simulink model "Stateflow_code"  (R2020a)
settings: Solver=ode5  StartTime=0.0  StopTime=inf  FixedStep=0.01  RelTol=1e-3
StopFcn:
  | clear con
model workspace (MAT data in the model file):
  A : Simulink.Signal (value not decoded)
undefined symbols (not defined in the file or in its folder): sigbuilder_block
libraries: simulink x10, simulink_extras x7, aerolibanimutils x1, powerlib_meascontrol x1, dspswit3 x1
(part 2 of 2)

== system Stateflow_code/Systemtest Simulation1/2_rot_mit_Deckel/luft_an ==
  Add : Sum
  Constant : Constant
  Constant1 : Constant  Value=-1
  Data Type Conversion : DataTypeConversion  OutDataTypeStr=boolean
  Delay : Delay  DelayLength=550
  Delay1 : Delay  DelayLength=750
  Out1 : Outport  VectorParamsAs1DForOutWhenUnconnected=off
  wires:
  Constant/1 -> Delay/1
  Constant1/1 -> Delay1/1
  Delay/1 -> Add/1
  Delay1/1 -> Add/2
  Add/1 -> Data Type Conversion/1
  Data Type Conversion/1 -> Out1/1

== system Stateflow_code/Systemtest Simulation1/2_rot_mit_Deckel/out5 ==
  Add : Sum
  Constant : Constant
  Constant1 : Constant  Value=-1
  Data Type Conversion : DataTypeConversion  OutDataTypeStr=boolean
  Delay : Delay  DelayLength=0
  Delay1 : Delay  DelayLength=0
  Out1 : Outport  VectorParamsAs1DForOutWhenUnconnected=off
  wires:
  Constant/1 -> Delay/1
  Constant1/1 -> Delay1/1
  Delay/1 -> Add/1
  Delay1/1 -> Add/2
  Add/1 -> Data Type Conversion/1
  Data Type Conversion/1 -> Out1/1

== system Stateflow_code/Systemtest Simulation1/2_rot_mit_Deckel/out6 ==
  Add : Sum
  Constant : Constant
  Constant1 : Constant  Value=-1
  Data Type Conversion : DataTypeConversion  OutDataTypeStr=boolean
  Delay : Delay  DelayLength=0
  Delay1 : Delay  DelayLength=0
  Out1 : Outport  VectorParamsAs1DForOutWhenUnconnected=off
  wires:
  Constant/1 -> Delay/1
  Constant1/1 -> Delay1/1
  Delay/1 -> Add/1
  Delay1/1 -> Add/2
  Add/1 -> Data Type Conversion/1
  Data Type Conversion/1 -> Out1/1

== system Stateflow_code/Systemtest Simulation1/2_rot_mit_Deckel/out7 ==
  Add : Sum
  Constant : Constant
  Constant1 : Constant  Value=-1
  Data Type Conversion : DataTypeConversion  OutDataTypeStr=boolean
  Delay : Delay  DelayLength=0
  Delay1 : Delay  DelayLength=0
  Out1 : Outport  VectorParamsAs1DForOutWhenUnconnected=off
  wires:
  Constant/1 -> Delay/1
  Constant1/1 -> Delay1/1
  Delay/1 -> Add/1
  Delay1/1 -> Add/2
  Add/1 -> Data Type Conversion/1
  Data Type Conversion/1 -> Out1/1

== system Stateflow_code/Systemtest Simulation1/2_rot_mit_Deckel/station_frei ==
  Add : Sum
  Constant : Constant
  Constant1 : Constant  Value=-1
  Data Type Conversion : DataTypeConversion  OutDataTypeStr=boolean
  Delay : Delay  DelayLength=0
  Delay1 : Delay  DelayLength=10
  Out1 : Outport  VectorParamsAs1DForOutWhenUnconnected=off
  wires:
  Constant/1 -> Delay/1
  Constant1/1 -> Delay1/1
  Delay/1 -> Add/1
  Delay1/1 -> Add/2
  Add/1 -> Data Type Conversion/1
  Data Type Conversion/1 -> Out1/1

== system Stateflow_code/Systemtest Simulation1/2_rot_mit_Deckel/zylinder_ausschieben ==
  Add : Sum
  Constant : Constant
  Constant1 : Constant  Value=-1
  Data Type Conversion : DataTypeConversion  OutDataTypeStr=boolean
  Delay : Delay  DelayLength=550
  Delay1 : Delay  DelayLength=620
  Out1 : Outport  VectorParamsAs1DForOutWhenUnconnected=off
  wires:
  Constant/1 -> Delay/1
  Constant1/1 -> Delay1/1
  Delay/1 -> Add/1
  Delay1/1 -> Add/2
  Add/1 -> Data Type Conversion/1
  Data Type Conversion/1 -> Out1/1

== system Stateflow_code/Systemtest Simulation1/2_rot_mit_Deckel/zylinder_entfernt_folge ==
  Add : Sum
  Constant : Constant
  Constant1 : Constant  Value=-1
  Data Type Conversion : DataTypeConversion  OutDataTypeStr=boolean
  Delay : Delay  DelayLength=1000
  Delay1 : Delay  DelayLength=1050
  Out1 : Outport  VectorParamsAs1DForOutWhenUnconnected=off
  wires:
  Constant/1 -> Delay/1
  Constant1/1 -> Delay1/1
  Delay/1 -> Add/1
  Delay1/1 -> Add/2
  Add/1 -> Data Type Conversion/1
  Data Type Conversion/1 -> Out1/1

== system Stateflow_code/Systemtest Simulation1/2_rot_mit_Deckel/zylinder_hoehe ==
  Add : Sum
  Constant : Constant  Value=28
  Constant1 : Constant  Value=-28
  Delay : Delay  DelayLength=50
  Delay1 : Delay  DelayLength=900
  Out1 : Outport  VectorParamsAs1DForOutWhenUnconnected=off
  wires:
  Constant/1 -> Delay/1
  Constant1/1 -> Delay1/1
  Delay/1 -> Add/1
  Delay1/1 -> Add/2
  Add/1 -> Out1/1

== system Stateflow_code/Systemtest Simulation1/2_rot_mit_Deckel/zylinder_platziert ==
  Add : Sum
  Constant : Constant
  Constant1 : Constant  Value=-1
  Data Type Conversion : DataTypeConversion  OutDataTypeStr=boolean
  Delay : Delay  DelayLength=0
  Delay1 : Delay  DelayLength=30
  Out1 : Outport  VectorParamsAs1DForOutWhenUnconnected=off
  wires:
  Constant/1 -> Delay/1
  Constant1/1 -> Delay1/1
  Delay/1 -> Add/1
  Delay1/1 -> Add/2
  Add/1 -> Data Type Conversion/1
  Data Type Conversion/1 -> Out1/1

== system Stateflow_code/Systemtest Simulation1/2_rot_mit_Deckel/zylinder_schwarz ==
  Add : Sum
  Constant : Constant
  Constant1 : Constant  Value=-1
  Data Type Conversion : DataTypeConversion  OutDataTypeStr=boolean
  Delay : Delay  DelayLength=0
  Delay1 : Delay  DelayLength=0
  Out1 : Outport  VectorParamsAs1DForOutWhenUnconnected=off
  wires:
  Constant/1 -> Delay/1
  Constant1/1 -> Delay1/1
  Delay/1 -> Add/1
  Delay1/1 -> Add/2
  Add/1 -> Data Type Conversion/1
  Data Type Conversion/1 -> Out1/1

== system Stateflow_code/Systemtest Simulation1/3_rot_ohne_Deckel/Signal Builder10 ==
  Demux : Demux  Tag=STV Demux  Outputs=8
      settings: DisplayOption=none
  FromWs : FromWorkspace  Tag=STV FromWs  VariableName=tuvar
      SigBuilderData=|
      | common.afterFinalStr = 'Extrapolate'
      | common.sampleTime = 0
      | dataSet.timeRange = [0 11]
      | dataSet.name = 'Group 1'
      | sbobj.Groups.Name = 'Group 1'
      | sbobj.Groups.Signals(1).Name = 'aufzug_abwaerts'
      | sbobj.Groups.Signals(1).XData = [0 5.5 5.5 10 10 11]
      | sbobj.Groups.Signals(1).YData = [0 0 1 1 0 0]
      | sbobj.Groups.Signals(2).Name = 'aufzug_aufwaerts'
      | sbobj.Groups.Signals(2).XData = [0 0.5 0.5 5 5 11]
      | sbobj.Groups.Signals(2).YData = [0 0 1 1 0 0]
      | sbobj.Groups.Signals(3).Name = 'zylinder_ausschieben'
      | sbobj.Groups.Signals(3).XData = [0 10 10 10.48 10.48 11]
      | sbobj.Groups.Signals(3).YData = [0 0 1 1 0 0]
      | sbobj.Groups.Signals(4).Name = 'luft_an'
      | sbobj.Groups.Signals(4).XData = [0 7.5 11]
      | sbobj.Groups.Signals(4).YData = [0 0 0]
      | sbobj.Groups.Signals(5).Name = 'Signal 5'
      | sbobj.Groups.Signals(5).XData = [0 11]
      | sbobj.Groups.Signals(5).YData = [0 0]
      | sbobj.Groups.Signals(6).Name = 'Signal 6'
      | sbobj.Groups.Signals(6).XData = [0 11]
      | sbobj.Groups.Signals(6).YData = [0 0]
      | sbobj.Groups.Signals(7).Name = 'Signal 7'
      | sbobj.Groups.Signals(7).XData = [0 11]
      | sbobj.Groups.Signals(7).YData = [0 0]
      | sbobj.Groups.Signals(8).Name = 'station_frei'
      | sbobj.Groups.Signals(8).XData = [0 0.1 0.1 11]
      | sbobj.Groups.Signals(8).YData = [1 1 0 0]
      | sbobj.Groups.TimeRange = [0 11]
  aufzug_abwaerts : Outport  Tag=STV Outport  VectorParamsAs1DForOutWhenUnconnected=off
  aufzug_aufwaerts : Outport  Tag=STV Outport  Port=2  VectorParamsAs1DForOutWhenUnconnected=off
  zylinder_ausschieben : Outport  Tag=STV Outport  Port=3  VectorParamsAs1DForOutWhenUnconnected=off
  luft_an : Outport  Tag=STV Outport  Port=4  VectorParamsAs1DForOutWhenUnconnected=off
  Signal 5 : Outport  Tag=STV Outport  Port=5  VectorParamsAs1DForOutWhenUnconnected=off
  Signal 6 : Outport  Tag=STV Outport  Port=6  VectorParamsAs1DForOutWhenUnconnected=off
  Signal 7 : Outport  Tag=STV Outport  Port=7  VectorParamsAs1DForOutWhenUnconnected=off
  station_frei : Outport  Tag=STV Outport  Port=8  VectorParamsAs1DForOutWhenUnconnected=off
  wires:
  Demux/1 -> aufzug_abwaerts/1
  FromWs/1 -> Demux/1
  Demux/2 -> aufzug_aufwaerts/1
  Demux/3 -> zylinder_ausschieben/1
  Demux/4 -> luft_an/1
  Demux/5 -> Signal 5/1
  Demux/6 -> Signal 6/1
  Demux/7 -> Signal 7/1
  Demux/8 -> station_frei/1

== system Stateflow_code/Systemtest Simulation1/3_rot_ohne_Deckel/Signal Builder4 ==
  Demux : Demux  Tag=STV Demux  Outputs=6
      settings: DisplayOption=none
  FromWs : FromWorkspace  Tag=STV FromWs  VariableName=tuvar
      SigBuilderData=|
      | common.afterFinalStr = 'Extrapolate'
      | common.sampleTime = 0
      | dataSet.timeRange = [0 11]
      | dataSet.name = 'Group 1'
      | sbobj.Groups.Name = 'Group 1'
      | sbobj.Groups.Signals(1).Name = 'zylinder_platziert'
      | sbobj.Groups.Signals(1).XData = [0 0.3 0.3 11]
      | sbobj.Groups.Signals(1).YData = [1 1 0 0]
      | sbobj.Groups.Signals(2).Name = 'zylinder_schwarz'
      | sbobj.Groups.Signals(2).XData = [0 11]
      | sbobj.Groups.Signals(2).YData = [0 0]
      | sbobj.Groups.Signals(3).Name = 'zylinder_hoehe'
      | sbobj.Groups.Signals(3).XData = [0 5 5 5.6 5.6 11]
      | sbobj.Groups.Signals(3).YData = [0 0 25 25 0 0]
      | sbobj.Groups.Signals(4).Name = 'arbeitsraum_frei'
      | sbobj.Groups.Signals(4).XData = [0 0.5 0.5 10 10 10.8 10.8 11]
      | sbobj.Groups.Signals(4).YData = [1 1 0 0 1 1 0 0]
      | sbobj.Groups.Signals(5).Name = 'zylinder_entfernt_folge'
      | sbobj.Groups.Signals(5).XData = [0 10 10.5 11]
      | sbobj.Groups.Signals(5).YData = [0 0 0 0]
      | sbobj.Groups.Signals(6).Name = 'folge_belegt'
      | sbobj.Groups.Signals(6).XData = [0 4 5.5 11]
      | sbobj.Groups.Signals(6).YData = [0 0 0 0]
      | sbobj.Groups.TimeRange = [0 11]
  zylinder_platziert : Outport  Tag=STV Outport  VectorParamsAs1DForOutWhenUnconnected=off
  zylinder_schwarz : Outport  Tag=STV Outport  Port=2  VectorParamsAs1DForOutWhenUnconnected=off
  zylinder_hoehe : Outport  Tag=STV Outport  Port=3  VectorParamsAs1DForOutWhenUnconnected=off
  arbeitsraum_frei : Outport  Tag=STV Outport  Port=4  VectorParamsAs1DForOutWhenUnconnected=off
  zylinder_entfernt_folge : Outport  Tag=STV Outport  Port=5  VectorParamsAs1DForOutWhenUnconnected=off
  folge_belegt : Outport  Tag=STV Outport  Port=6  VectorParamsAs1DForOutWhenUnconnected=off
  wires:
  Demux/1 -> zylinder_platziert/1
  FromWs/1 -> Demux/1
  Demux/2 -> zylinder_schwarz/1
  Demux/3 -> zylinder_hoehe/1
  Demux/4 -> arbeitsraum_frei/1
  Demux/5 -> zylinder_entfernt_folge/1
  Demux/6 -> folge_belegt/1

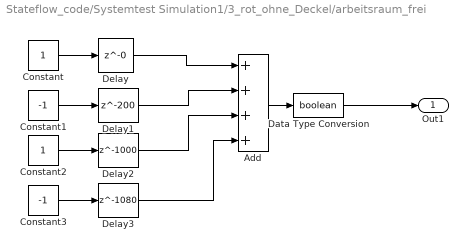
== system Stateflow_code/Systemtest Simulation1/3_rot_ohne_Deckel/arbeitsraum_frei ==
  Add : Sum  Inputs=++++
  Constant : Constant
  Constant1 : Constant  Value=-1
  Constant2 : Constant
  Constant3 : Constant  Value=-1
  Data Type Conversion : DataTypeConversion  OutDataTypeStr=boolean
  Delay : Delay  DelayLength=0
  Delay1 : Delay  DelayLength=200
  Delay2 : Delay  DelayLength=1000
  Delay3 : Delay  DelayLength=1080
  Out1 : Outport  VectorParamsAs1DForOutWhenUnconnected=off
  wires:
  Constant/1 -> Delay/1
  Constant1/1 -> Delay1/1
  Delay/1 -> Add/1
  Delay1/1 -> Add/2
  Add/1 -> Data Type Conversion/1
  Data Type Conversion/1 -> Out1/1
  Constant2/1 -> Delay2/1
  Delay2/1 -> Add/3
  Constant3/1 -> Delay3/1
  Delay3/1 -> Add/4

== system Stateflow_code/Systemtest Simulation1/3_rot_ohne_Deckel/aufzug_abwaerts ==
  Add : Sum
  Constant : Constant
  Constant1 : Constant  Value=-1
  Data Type Conversion : DataTypeConversion  OutDataTypeStr=boolean
  Delay : Delay  DelayLength=550
  Delay1 : Delay  DelayLength=1000
  Out1 : Outport  VectorParamsAs1DForOutWhenUnconnected=off
  wires:
  Constant/1 -> Delay/1
  Constant1/1 -> Delay1/1
  Delay/1 -> Add/1
  Delay1/1 -> Add/2
  Add/1 -> Data Type Conversion/1
  Data Type Conversion/1 -> Out1/1

== system Stateflow_code/Systemtest Simulation1/3_rot_ohne_Deckel/aufzug_aufwaerts ==
  Add : Sum
  Constant : Constant
  Constant1 : Constant  Value=-1
  Data Type Conversion : DataTypeConversion  OutDataTypeStr=boolean
  Delay : Delay  DelayLength=50
  Delay1 : Delay  DelayLength=500
  Out1 : Outport  VectorParamsAs1DForOutWhenUnconnected=off
  wires:
  Constant/1 -> Delay/1
  Constant1/1 -> Delay1/1
  Delay/1 -> Add/1
  Delay1/1 -> Add/2
  Add/1 -> Data Type Conversion/1
  Data Type Conversion/1 -> Out1/1

== system Stateflow_code/Systemtest Simulation1/3_rot_ohne_Deckel/folge_belegt ==
  Constant : Constant  Value=0
  Data Type Conversion : DataTypeConversion  OutDataTypeStr=boolean
  Out1 : Outport  VectorParamsAs1DForOutWhenUnconnected=off
  wires:
  Constant/1 -> Data Type Conversion/1
  Data Type Conversion/1 -> Out1/1

== system Stateflow_code/Systemtest Simulation1/3_rot_ohne_Deckel/luft_an ==
  Add : Sum
  Constant : Constant
  Constant1 : Constant  Value=-1
  Data Type Conversion : DataTypeConversion  OutDataTypeStr=boolean
  Delay : Delay  DelayLength=0
  Delay1 : Delay  DelayLength=0
  Out1 : Outport  VectorParamsAs1DForOutWhenUnconnected=off
  wires:
  Constant/1 -> Delay/1
  Constant1/1 -> Delay1/1
  Delay/1 -> Add/1
  Delay1/1 -> Add/2
  Add/1 -> Data Type Conversion/1
  Data Type Conversion/1 -> Out1/1

== system Stateflow_code/Systemtest Simulation1/3_rot_ohne_Deckel/out5 ==
  Add : Sum
  Constant : Constant
  Constant1 : Constant  Value=-1
  Data Type Conversion : DataTypeConversion  OutDataTypeStr=boolean
  Delay : Delay  DelayLength=0
  Delay1 : Delay  DelayLength=0
  Out1 : Outport  VectorParamsAs1DForOutWhenUnconnected=off
  wires:
  Constant/1 -> Delay/1
  Constant1/1 -> Delay1/1
  Delay/1 -> Add/1
  Delay1/1 -> Add/2
  Add/1 -> Data Type Conversion/1
  Data Type Conversion/1 -> Out1/1

== system Stateflow_code/Systemtest Simulation1/3_rot_ohne_Deckel/out6 ==
  Add : Sum
  Constant : Constant
  Constant1 : Constant  Value=-1
  Data Type Conversion : DataTypeConversion  OutDataTypeStr=boolean
  Delay : Delay  DelayLength=0
  Delay1 : Delay  DelayLength=0
  Out1 : Outport  VectorParamsAs1DForOutWhenUnconnected=off
  wires:
  Constant/1 -> Delay/1
  Constant1/1 -> Delay1/1
  Delay/1 -> Add/1
  Delay1/1 -> Add/2
  Add/1 -> Data Type Conversion/1
  Data Type Conversion/1 -> Out1/1

== system Stateflow_code/Systemtest Simulation1/3_rot_ohne_Deckel/out7 ==
  Add : Sum
  Constant : Constant
  Constant1 : Constant  Value=-1
  Data Type Conversion : DataTypeConversion  OutDataTypeStr=boolean
  Delay : Delay  DelayLength=0
  Delay1 : Delay  DelayLength=0
  Out1 : Outport  VectorParamsAs1DForOutWhenUnconnected=off
  wires:
  Constant/1 -> Delay/1
  Constant1/1 -> Delay1/1
  Delay/1 -> Add/1
  Delay1/1 -> Add/2
  Add/1 -> Data Type Conversion/1
  Data Type Conversion/1 -> Out1/1

== system Stateflow_code/Systemtest Simulation1/3_rot_ohne_Deckel/station_frei ==
  Add : Sum
  Constant : Constant
  Constant1 : Constant  Value=-1
  Data Type Conversion : DataTypeConversion  OutDataTypeStr=boolean
  Delay : Delay  DelayLength=0
  Delay1 : Delay  DelayLength=10
  Out1 : Outport  VectorParamsAs1DForOutWhenUnconnected=off
  wires:
  Constant/1 -> Delay/1
  Constant1/1 -> Delay1/1
  Delay/1 -> Add/1
  Delay1/1 -> Add/2
  Add/1 -> Data Type Conversion/1
  Data Type Conversion/1 -> Out1/1

== system Stateflow_code/Systemtest Simulation1/3_rot_ohne_Deckel/zylinder_ausschieben ==
  Add : Sum
  Constant : Constant
  Constant1 : Constant  Value=-1
  Data Type Conversion : DataTypeConversion  OutDataTypeStr=boolean
  Delay : Delay  DelayLength=1000
  Delay1 : Delay  DelayLength=1050
  Out1 : Outport  VectorParamsAs1DForOutWhenUnconnected=off
  wires:
  Constant/1 -> Delay/1
  Constant1/1 -> Delay1/1
  Delay/1 -> Add/1
  Delay1/1 -> Add/2
  Add/1 -> Data Type Conversion/1
  Data Type Conversion/1 -> Out1/1

== system Stateflow_code/Systemtest Simulation1/3_rot_ohne_Deckel/zylinder_entfernt_folge ==
  Add : Sum
  Constant : Constant
  Constant1 : Constant  Value=-1
  Data Type Conversion : DataTypeConversion  OutDataTypeStr=boolean
  Delay : Delay  DelayLength=0
  Delay1 : Delay  DelayLength=0
  Out1 : Outport  VectorParamsAs1DForOutWhenUnconnected=off
  wires:
  Constant/1 -> Delay/1
  Constant1/1 -> Delay1/1
  Delay/1 -> Add/1
  Delay1/1 -> Add/2
  Add/1 -> Data Type Conversion/1
  Data Type Conversion/1 -> Out1/1

== system Stateflow_code/Systemtest Simulation1/3_rot_ohne_Deckel/zylinder_hoehe ==
  Add : Sum
  Constant : Constant  Value=25
  Constant1 : Constant  Value=-25
  Delay : Delay  DelayLength=50
  Delay1 : Delay  DelayLength=900
  Out1 : Outport  VectorParamsAs1DForOutWhenUnconnected=off
  wires:
  Constant/1 -> Delay/1
  Constant1/1 -> Delay1/1
  Delay/1 -> Add/1
  Delay1/1 -> Add/2
  Add/1 -> Out1/1

== system Stateflow_code/Systemtest Simulation1/3_rot_ohne_Deckel/zylinder_platziert ==
  Add : Sum
  Constant : Constant
  Constant1 : Constant  Value=-1
  Data Type Conversion : DataTypeConversion  OutDataTypeStr=boolean
  Delay : Delay  DelayLength=0
  Delay1 : Delay  DelayLength=30
  Out1 : Outport  VectorParamsAs1DForOutWhenUnconnected=off
  wires:
  Constant/1 -> Delay/1
  Constant1/1 -> Delay1/1
  Delay/1 -> Add/1
  Delay1/1 -> Add/2
  Add/1 -> Data Type Conversion/1
  Data Type Conversion/1 -> Out1/1

== system Stateflow_code/Systemtest Simulation1/3_rot_ohne_Deckel/zylinder_schwarz ==
  Add : Sum
  Constant : Constant
  Constant1 : Constant  Value=-1
  Data Type Conversion : DataTypeConversion  OutDataTypeStr=boolean
  Delay : Delay  DelayLength=0
  Delay1 : Delay  DelayLength=0
  Out1 : Outport  VectorParamsAs1DForOutWhenUnconnected=off
  wires:
  Constant/1 -> Delay/1
  Constant1/1 -> Delay1/1
  Delay/1 -> Add/1
  Delay1/1 -> Add/2
  Add/1 -> Data Type Conversion/1
  Data Type Conversion/1 -> Out1/1

== stateflow chart Stateflow_code/Pruefen_Angabe ==
  state With_Lid
    state Standby_withLid
      en: step = 11;
      en: t = clock;
    state lift_down_withLid
      en: step = 10;
      en: Aufzug_abwaerts = true;
      ex: Aufzug_abwaerts = false;
    state air_off
      en: step = 9;
      en: Luft_an = false;
    state cylinder_retracted_withLid
      en: step = 8;
      en: Zylinder_ausschieben = false;
      en: t = clock;
    state cylinder_extension_withLid
      en: step = 7;
      en: Zylinder_ausschieben = true;
      en: t = clock;
      en: Luft_an = true;
    lift_down_withLid -> Standby_withLid : [Aufzug_unten == true]
    air_off -> lift_down_withLid : [(Zylinder_eingefahren==1)]
    cylinder_retracted_withLid -> air_off : [(clock-1.5)>=t]
    cylinder_extension_withLid -> cylinder_retracted_withLid : [(clock-0.5)>=t]
    (default) -> cylinder_extension_withLid
  state Without_Lid
    state cylinder_retracted_withoutLid
      en: step = 6;
      en: Zylinder_ausschieben = false;
    state cylinder_extension_withoutLid
      en: step = 5;
      en: Zylinder_ausschieben = true;
      en: t = clock;
    state Standby_withoutLid
      en: step = 11;
      en: t = clock;
    state lift_down_withoutLid
      en: step = 4;
      en: Aufzug_abwaerts = true;
      ex: Aufzug_abwaerts = false;
    cylinder_extension_withoutLid -> cylinder_retracted_withoutLid : [(clock-0.5)>=t]
    Standby_withoutLid -> cylinder_extension_withoutLid : [(clock-0.5)>=t]
    lift_down_withoutLid -> Standby_withoutLid : [(Aufzug_unten==true)]
    (default) -> lift_down_withoutLid
  state initial_states
    en: step = 1;
    en: Zylinder_ausschieben = false;
    en: Luft_an = false;
    en: Station_frei = false;
    en: out4 = false;
    en: out5 = false;
    en: out6 = false;
  state ask_for_workpiece
    en: step = 2;
    en: Station_frei = true;
    ex: Station_frei = false;
  state Standby_upward
    en: step = 11;
    en: t = clock;
  state lift_up
    en: step = 3;
    en: Aufzug_aufwaerts = true;
    ex: Aufzug_aufwaerts = false;
  state Standby_measure
    en: step = 11;
    en: t = clock;
  Standby_withLid -> ask_for_workpiece : [(clock-0.5)>=t]
  (default) -> initial_states
  cylinder_retracted_withoutLid -> ask_for_workpiece : [(Zylinder_eingefahren==true)]
  initial_states -> ask_for_workpiece : [(Werkstueck_vorhanden==false) && (Aufzug_unten==true)]
  ask_for_workpiece -> Standby_upward : [(Werkstueck_vorhanden==true)]
  Standby_upward -> lift_up : [(Arbeitsraum_frei==true) && (clock - 0.5)>=t]
  lift_up -> Standby_measure : [(Aufzug_oben==true)]
  Standby_measure -> (junction 89) : [(clock-1)>=t]
  (junction 89) -> Without_Lid [order 2] : [(Hoehe_ok==Werkstueck_nicht_schwarz)]
  (junction 89) -> With_Lid [order 1] : [(Hoehe_ok~=Werkstueck_nicht_schwarz) && (Folgestation_belegt==false)]
  data: Aufzug_abwaerts output; Werkstueck_vorhanden input; Aufzug_aufwaerts output; Zylinder_ausschieben output; Luft_an output; out4 output; out5 output; out6 output; Station_frei output; step output; Werkstueck_nicht_schwarz input; Arbeitsraum_frei input; Hoehe_ok input; Aufzug_oben input; Aufzug_unten input; Zylinder_eingefahren input; Folgestation_belegt input; clock input; t local
